simulink model "SIM_6DOF_completo_qnathy_comparaPeixoto"  (R2021b)
settings: Solver=FixedStepAuto  StartTime=0.0  StopTime=D.Tfim  FixedStep=0.001  MaxStep=0.001  RelTol=1e-3
undefined symbols (not defined in the file): c, D, dados, desv_emp, erro, F, Light, M, MIL, Newton, Raphson, wind
libraries: aerolibasang x7, sharedutil x3, aerolibwind2 x3, shared6dof x2, aerolibanim x1, aerolibatmos2 x1, simulink x1, dspmtrx3 x1, sharedtransform x1
(part 2 of 2)

== system SIM_6DOF_completo_qnathy_comparaPeixoto/Dinamica 6DOF/Aerodinamica/Subsystem2/If Action Subsystem ==
  In1 : Inport
  Action Port : ActionPort  ActionPortLabel=if(u1 > 2500)
  CA_airbrake : Lookup_n-D  NumberOfTableDimensions=4  BreakpointsForDimension1=dados.phif  BreakpointsForDimension2=dados.mach  BreakpointsForDimension3=dados.alpha  BreakpointsForDimension4=dados.cg  BreakpointsForDimension5=dados.phif  BreakpointsForDimension6=dados.mach  BreakpointsForDimension7=dados.alpha  BreakpointsForDimension8=dados.cg  Table=M.CA  ExtrapMethod=Clip  InternalRulePriority=Speed  RndMeth=Simplest  InputSameDT=on
      settings: InputPortMap=u0,u1,u2,u3
  Demux3 : Demux  Outputs=3
  Terminator7 : Terminator
  Terminator8 : Terminator
  Out1 : Outport
  wires:
  [mach] -> CA_airbrake/2
  Demux3/1 -> CA_airbrake/4
  [phi] -> CA_airbrake/1
  [CG] -> Demux3/1
  [alfatotal] -> CA_airbrake/3
  Demux3/3 -> Terminator8/1
  CA_airbrake/1 -> Out1/1
  Demux3/2 -> Terminator7/1

== system SIM_6DOF_completo_qnathy_comparaPeixoto/Dinamica 6DOF/Aerodinamica/Subsystem2/If Action Subsystem1 ==
  In1 : Inport
  Action Port : ActionPort  ActionPortLabel=else
  CA1 : Lookup_n-D  NumberOfTableDimensions=4  BreakpointsForDimension1=dados.phif  BreakpointsForDimension2=dados.mach  BreakpointsForDimension3=dados.alpha  BreakpointsForDimension4=dados.cg  BreakpointsForDimension5=dados.phif  BreakpointsForDimension6=dados.mach  BreakpointsForDimension7=dados.alpha  BreakpointsForDimension8=dados.cg  Table=M.CA  ExtrapMethod=Clip  InternalRulePriority=Speed  RndMeth=Simplest  InputSameDT=on
      settings: InputPortMap=u0,u1,u2,u3
  Demux1 : Demux  Outputs=3
  Terminator1 : Terminator
  Terminator2 : Terminator
  Out1 : Outport
  wires:
  [phi] -> CA1/1
  Demux1/3 -> Terminator2/1
  [CG] -> Demux1/1
  CA1/1 -> Out1/1
  [alfatotal] -> CA1/3
  Demux1/2 -> Terminator1/1
  Demux1/1 -> CA1/4
  [mach] -> CA1/2

== system SIM_6DOF_completo_qnathy_comparaPeixoto/Dinamica 6DOF/Aerodinamica/Subsystem8/Subsystem2 ==
  Vb : Inport
  Airspeed : Sqrt  AlgorithmType=Newton-Raphson  SaturateOnIntegerOverflow=on
  Incidence : Trigonometry  Operator=atan2
  Incidence1 : Trigonometry  Operator=atan2
  Subsystem : aerolibasang/Incidence, Sideslip, & Airspeed/Subsystem  SystemSampleTime=-1  VariantActivationTime=update diagram  Latency=0  AutoFrameSizeCalculation=off
      settings: SourceProductBaseCode=AE
  Subsystem1 : aerolibasang/Incidence, Sideslip, & Airspeed/Subsystem1  SystemSampleTime=-1  VariantActivationTime=update diagram  Latency=0  AutoFrameSizeCalculation=off
      settings: SourceProductBaseCode=AE
  dot : aerolibasang/Incidence, Sideslip, & Airspeed/dot  SystemSampleTime=-1  VariantActivationTime=update diagram  Latency=0  AutoFrameSizeCalculation=off
      settings: SourceProductBaseCode=AE
  Alfa : Outport  VectorParamsAs1DForOutWhenUnconnected=off
  Beta : Outport  Port=2  VectorParamsAs1DForOutWhenUnconnected=off
  V : Outport  Port=3  VectorParamsAs1DForOutWhenUnconnected=off
  wires:
  Subsystem1/1 -> Incidence1/1
  Incidence/1 -> Alfa/1
  Subsystem/1 -> Incidence/1
  dot/1 -> Airspeed/1
  Incidence1/1 -> Beta/1
  Subsystem/2 -> Incidence1/2, Incidence/2
  Vb/1 -> Subsystem1/1, dot/1, Subsystem/1
  Airspeed/1 -> V/1

== system SIM_6DOF_completo_qnathy_comparaPeixoto/Dinamica 6DOF/Aerodinamica/Subsystem8/Subsystem6 ==
  d : Inport
  Velocity : Inport  Port=2
  Divide : Product  Inputs=*/
  d/(2V) : Gain  Gain=1/2  SaturateOnIntegerOverflow=on  OutDataTypeStr=Inherit: Same as input  ParamDataTypeStr=Inherit: Same as input
  dot : aerolibasang/Dynamic Pressure/dot  SystemSampleTime=-1  VariantActivationTime=update diagram  Latency=0  AutoFrameSizeCalculation=off
      settings: SourceProductBaseCode=AE
  vt : Sqrt  AlgorithmType=Newton-Raphson  SaturateOnIntegerOverflow=on
  d2V : Outport  InitialOutput=0  VectorParamsAs1DForOutWhenUnconnected=off
  wires:
  d/(2V)/1 -> d2V/1
  Velocity/1 -> dot/1
  Divide/1 -> d/(2V)/1
  dot/1 -> vt/1
  d/1 -> Divide/1
  vt/1 -> Divide/2
